simulink library "DQN_Lib (conflicted copy 2023-11-25 154811)"  (R2023b)
settings: Solver=VariableStepAuto  StartTime=0.0  StopTime=10.0  RelTol=1e-3
undefined symbols (not defined in the file): FreqRad, HrmOrd, Init, La, N, R, Ra, TimeStep, Ts, Ts_dqn, Ws
libraries: $bdroot x4, spsMeanVariableFrequencyLib x4, eeTransforms x3, spsabctodq0Lib x2, spsAlphaBetaZerotodq0Lib x1
(part 2 of 8)

== system DQN_Lib (conflicted copy 2023-11-25 154811)/Int_DQN ==
  X_DQN : Inport
  Demux : Demux  Outputs=6
  Int_d_2N_2 : MATLAB Function  TreatAsAtomicUnit=on  mask{N=HrmOrd, dt=TimeStep, w=FreqRad, EMT=EMT, InitInt=Init, chkHrmLst=chkHrmLst, HrmLst=HrmLst}
      mask prompts: N "Order number:"; dt "Time step (s):"; w "Angular frequency (1/rad):"; InitInt "Initial conditions [6x1]:"; chkHrmLst "Only selected harmonics"; HrmLst "Harmonic list:"
  Mux51 : Mux  Inputs=[(1)*HrmOrd+1,(1)*HrmOrd+1,(1)*HrmOrd+1,(1)*HrmOrd+1,(1)*HrmOrd+1,(1)*HrmOrd+1]
  Z_DQN : Outport
  wires:
  X_DQN/1 -> Demux/1
  Mux51/1 -> Z_DQN/1
  Demux/3 -> Int_d_2N_2/3(Xdz)
  Demux/2 -> Int_d_2N_2/2(Xdn)
  Demux/4 -> Int_d_2N_2/4(Xqp)
  Demux/1 -> Int_d_2N_2/1(Xdp)
  Demux/5 -> Int_d_2N_2/5(Xqn)
  Demux/6 -> Int_d_2N_2/6(Xqz)
  Int_d_2N_2/3(Zdz) -> Mux51/3
  Int_d_2N_2/2(Zdn) -> Mux51/2
  Int_d_2N_2/4(Zqp) -> Mux51/4
  Int_d_2N_2/1(Zdp) -> Mux51/1
  Int_d_2N_2/5(Zqn) -> Mux51/5
  Int_d_2N_2/6(Zqz) -> Mux51/6

== system DQN_Lib (conflicted copy 2023-11-25 154811)/Int_DQN_fdbk ==
  X_DQN : Inport
  Demux : Demux  Outputs=6
  Int_d_2N_2 : MATLAB Function  TreatAsAtomicUnit=on  mask{N=HrmOrd, dt=TimeStep, w=FreqRad, SW=swFeed, R=R, iL=iL}
      mask prompts: N "Order number:"; dt "Time step (s):"; w "Angular frequency (1/rad):"; SW "Enable feedback"; R "Feedback parameter (Kr):"; iL "Integrator parameter (Kl):"
  Mux51 : Mux  Inputs=[(1)*HrmOrd+1,(1)*HrmOrd+1,(1)*HrmOrd+1,(1)*HrmOrd+1,(1)*HrmOrd+1,(1)*HrmOrd+1]
  Z_DQN : Outport
  wires:
  Int_d_2N_2/6(Zqz) -> Mux51/6
  Int_d_2N_2/5(Zqn) -> Mux51/5
  Int_d_2N_2/1(Zdp) -> Mux51/1
  Int_d_2N_2/4(Zqp) -> Mux51/4
  Int_d_2N_2/2(Zdn) -> Mux51/2
  Int_d_2N_2/3(Zdz) -> Mux51/3
  Demux/6 -> Int_d_2N_2/6(Xqz)
  Demux/5 -> Int_d_2N_2/5(Xqn)
  Demux/1 -> Int_d_2N_2/1(Xdp)
  Demux/4 -> Int_d_2N_2/4(Xqp)
  Demux/2 -> Int_d_2N_2/2(Xdn)
  Demux/3 -> Int_d_2N_2/3(Xdz)
  Mux51/1 -> Z_DQN/1
  X_DQN/1 -> Demux/1

== system DQN_Lib (conflicted copy 2023-11-25 154811)/MatDemux ==
  In1 : Inport
  Sel1 : Selector  NumberOfDimensions=2  InputPortWidth=3  IndexOptions=Select all,Index vector (dialog)  Indices=1,1:6  OutputSizes=1
  Sel2 : Selector  NumberOfDimensions=2  InputPortWidth=3  IndexOptions=Select all,Index vector (dialog)  Indices=1,7:12  OutputSizes=1
  Sel3 : Selector  NumberOfDimensions=2  InputPortWidth=3  IndexOptions=Select all,Index vector (dialog)  Indices=1,13:18  OutputSizes=1
  Out1 : Outport
  Out2 : Outport  Port=2
  Out3 : Outport  Port=3
  wires:
  In1/1 -> Sel1/1, Sel2/1, Sel3/1
  Sel1/1 -> Out1/1
  Sel2/1 -> Out2/1
  Sel3/1 -> Out3/1

== system DQN_Lib (conflicted copy 2023-11-25 154811)/MatMux ==
  In1 : Inport
  In2 : Inport  Port=2
  In3 : Inport  Port=3
  Mux : Concatenate  NumInputs=3  Mode=Multidimensional array  ConcatenateDimension=2
  Out1 : Outport
  wires:
  In1/1 -> Mux/1
  In2/1 -> Mux/2
  In3/1 -> Mux/3
  Mux/1 -> Out1/1

== system DQN_Lib (conflicted copy 2023-11-25 154811)/Mult_DQN ==
  X_DQN : Inport
  Y_DQN : Inport  Port=2
  DQn (Full)10 : MATLAB Function  TreatAsAtomicUnit=on  mask{N=HrmOrd, HrmDbl=HrmDbl, chkHrmLst=chkHrmLst, HrmLstX=HrmLstX, HrmLstY=HrmLstY}
      mask prompts: N "Harmonic order:"; HrmDbl "Double Harmonic"; chkHrmLst "Only specific harmonics:"; HrmLstX "Harmonic list X:"; HrmLstY "Harmonic list Y:"
  Demux : Demux  Outputs=6
  Demux1 : Demux  Outputs=6
  Mux51 : Mux  Inputs=[(HrmDbl+1)*HrmOrd+1,(HrmDbl+1)*HrmOrd+1,(HrmDbl+1)*HrmOrd+1,(HrmDbl+1)*HrmOrd+1,(HrmDbl+1)*HrmOrd+1,(HrmDbl+1)*HrmOrd+1]
  Z_DQN : Outport
  wires:
  X_DQN/1 -> Demux/1
  Y_DQN/1 -> Demux1/1
  Mux51/1 -> Z_DQN/1
  Demux/1 -> DQn (Full)10/1(Xdp)
  Demux/2 -> DQn (Full)10/2(Xdn)
  Demux/3 -> DQn (Full)10/3(Xdz)
  Demux/4 -> DQn (Full)10/4(Xqp)
  Demux/5 -> DQn (Full)10/5(Xqn)
  Demux/6 -> DQn (Full)10/6(Xqz)
  Demux1/1 -> DQn (Full)10/7(Ydp)
  Demux1/2 -> DQn (Full)10/8(Ydn)
  Demux1/3 -> DQn (Full)10/9(Ydz)
  Demux1/4 -> DQn (Full)10/10(Yqp)
  Demux1/5 -> DQn (Full)10/11(Yqn)
  Demux1/6 -> DQn (Full)10/12(Yqz)
  DQn (Full)10/3(Zdz) -> Mux51/3
  DQn (Full)10/2(Zdn) -> Mux51/2
  DQn (Full)10/4(Zqp) -> Mux51/4
  DQn (Full)10/1(Zdp) -> Mux51/1
  DQn (Full)10/5(Zqn) -> Mux51/5
  DQn (Full)10/6(Zqz) -> Mux51/6

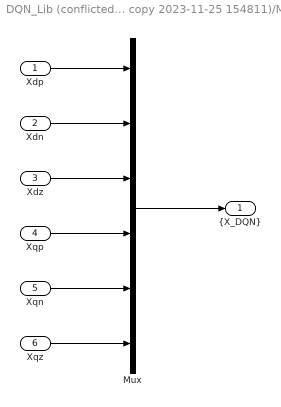
== system DQN_Lib (conflicted copy 2023-11-25 154811)/Mux ==
  Xdp : Inport
  Xdn : Inport  Port=2
  Xdz : Inport  Port=3
  Xqp : Inport  Port=4
  Xqn : Inport  Port=5
  Xqz : Inport  Port=6
  Mux : Mux  Inputs=[N+1, N+1, N+1, N+1, N+1, N+1]
  "{X_DQN}" : Outport
  wires:
  Mux/1 -> "{X_DQN}"/1
  Xdp/1 -> Mux/1
  Xdn/1 -> Mux/2
  Xdz/1 -> Mux/3
  Xqp/1 -> Mux/4
  Xqn/1 -> Mux/5
  Xqz/1 -> Mux/6

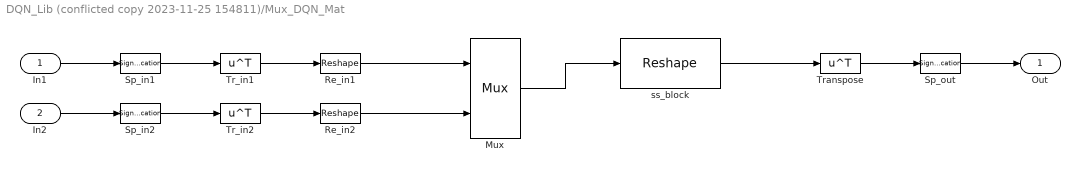
== system DQN_Lib (conflicted copy 2023-11-25 154811)/Mux_DQN_Mat ==
  In1 : Inport
  In2 : Inport  Port=2
  Mux : Mux  Inputs=[6,6]
  Re_in1 : Reshape
  Re_in2 : Reshape
  Sp_in1 : SignalSpecification  Dimensions=[1,6]
  Sp_in2 : SignalSpecification  Dimensions=[1,6]
  Sp_out : SignalSpecification  Dimensions=[2,6]
  Tr_in1 : Math  Operator=transpose
  Tr_in2 : Math  Operator=transpose
  Transpose : Math  Operator=transpose
  ss_block : Reshape  OutputDimensionality=Customize  OutputDimensions=[6,2*(1)]
  Out : Outport
  wires:
  In1/1 -> Sp_in1/1
  Sp_in1/1 -> Tr_in1/1
  Tr_in1/1 -> Re_in1/1
  Re_in1/1 -> Mux/1
  In2/1 -> Sp_in2/1
  Sp_in2/1 -> Tr_in2/1
  Tr_in2/1 -> Re_in2/1
  Re_in2/1 -> Mux/2
  Mux/1 -> ss_block/1
  ss_block/1 -> Transpose/1
  Transpose/1 -> Sp_out/1
  Sp_out/1 -> Out/1

== system DQN_Lib (conflicted copy 2023-11-25 154811)/Mux_DQNc_Mat ==
  In1 : Inport
  In2 : Inport  Port=2
  Mux : Concatenate  Mode=Multidimensional array
  Out1 : Outport
  wires:
  In1/1 -> Mux/1
  In2/1 -> Mux/2
  Mux/1 -> Out1/1

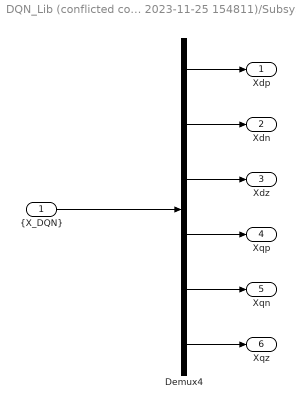
== system DQN_Lib (conflicted copy 2023-11-25 154811)/Subsystem ==
  "{X_DQN}" : Inport
  Demux4 : Demux  Outputs=[N+1, N+1, N+1, N+1, N+1, N+1]
  Xdp : Outport
  Xdn : Outport  Port=2
  Xdz : Outport  Port=3
  Xqp : Outport  Port=4
  Xqn : Outport  Port=5
  Xqz : Outport  Port=6
  wires:
  "{X_DQN}"/1 -> Demux4/1
  Demux4/1 -> Xdp/1
  Demux4/2 -> Xdn/1
  Demux4/3 -> Xdz/1
  Demux4/4 -> Xqp/1
  Demux4/5 -> Xqn/1
  Demux4/6 -> Xqz/1

== system DQN_Lib (conflicted copy 2023-11-25 154811)/Subsystem1 ==
  abc : Inport
  th : Inport  Port=2
  DQN Mux : MATLAB Function  TreatAsAtomicUnit=on  mask{N=1}
      mask prompts: N "Harmonic order:"
  Mux : Mux  Inputs=[1, 1, 1, 1, 1, 1]
  Mux1 : Mux  Inputs=2
  abc-->DQN : $bdroot/abc-->DQN  H=HrmOrd  f=Freq  Ts=Ts
  DQN : Outport
  wires:
  th/1 -> abc-->DQN/2
  abc/1 -> abc-->DQN/1
  abc-->DQN/2 -> Mux/1
  abc-->DQN/3 -> Mux/2
  abc-->DQN/4 -> Mux/3
  abc-->DQN/5 -> Mux/4
  abc-->DQN/6 -> Mux/5
  abc-->DQN/7 -> Mux/6
  DQN Mux/1(y) -> DQN/1
  abc-->DQN/1 -> Mux1/1
  Mux1/1 -> DQN Mux/1(u)
  Mux/1 -> Mux1/2

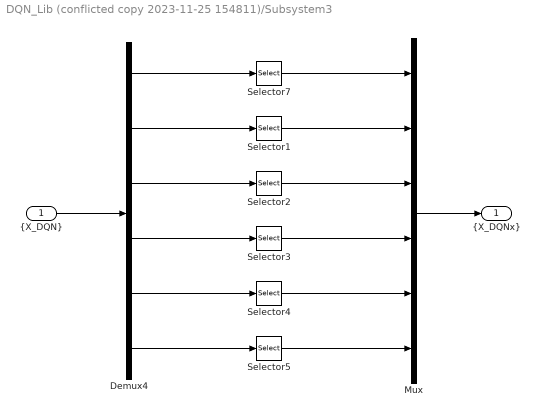
== system DQN_Lib (conflicted copy 2023-11-25 154811)/Subsystem3 ==
  "{X_DQN}" : Inport
  Demux4 : Demux  Outputs=[HOI+1,HOI+1,HOI+1,HOI+1,HOI+1,HOI+1]
  Mux : Mux  Inputs=[HOO+1,HOO+1,HOO+1,HOO+1,HOO+1,HOO+1]
  Selector{1..5,7} (6 alike) : Selector  InputPortWidth=HOI+1  IndexOptions=Index vector (dialog)  Indices=[1:HOO+1]  OutputSizes=1
  "{X_DQNx}" : Outport
  wires:
  "{X_DQN}"/1 -> Demux4/1
  Mux/1 -> "{X_DQNx}"/1
  Selector7/1 -> Mux/1
  Demux4/1 -> Selector7/1
  Selector1/1 -> Mux/2
  Demux4/2 -> Selector1/1
  Demux4/3 -> Selector2/1
  Selector2/1 -> Mux/3
  Demux4/4 -> Selector3/1
  Selector3/1 -> Mux/4
  Demux4/5 -> Selector4/1
  Selector4/1 -> Mux/5
  Demux4/6 -> Selector5/1
  Selector5/1 -> Mux/6

== system DQN_Lib (conflicted copy 2023-11-25 154811)/Subsystem4 ==
  In1 : Inport
  In2 : Inport  Port=2
  Demux : Demux  Outputs=6
  S-Function : S-Function  FunctionName=sDQNabc  SFunctionDeploymentMode=off  EnableBusSupport=off
  Out1 : Outport
  wires:
  Demux/5 -> S-Function/5
  Demux/4 -> S-Function/4
  Demux/6 -> S-Function/6
  Demux/2 -> S-Function/2
  S-Function/1 -> Out1/1
  Demux/1 -> S-Function/1
  Demux/3 -> S-Function/3
  In2/1 -> S-Function/7
  In1/1 -> Demux/1

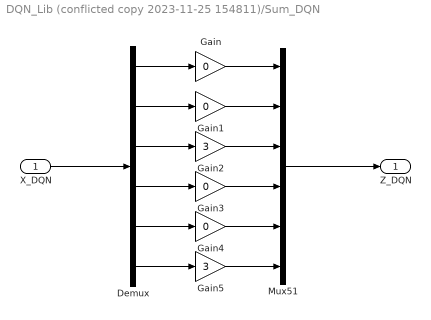
== system DQN_Lib (conflicted copy 2023-11-25 154811)/Sum_DQN ==
  X_DQN : Inport
  Demux : Demux  Outputs=[(1)*HrmOrd+1,(1)*HrmOrd+1,(1)*HrmOrd+1,(1)*HrmOrd+1,(1)*HrmOrd+1,(1)*HrmOrd+1]
  Gain{,1,3..4} (4 alike) : Gain  Gain=0
  Gain2 : Gain  Gain=3
  Gain5 : Gain  Gain=3
  Mux51 : Mux  Inputs=[(1)*HrmOrd+1,(1)*HrmOrd+1,(1)*HrmOrd+1,(1)*HrmOrd+1,(1)*HrmOrd+1,(1)*HrmOrd+1]
  Z_DQN : Outport
  wires:
  Mux51/1 -> Z_DQN/1
  X_DQN/1 -> Demux/1
  Gain/1 -> Mux51/1
  Demux/1 -> Gain/1
  Demux/2 -> Gain1/1
  Gain1/1 -> Mux51/2
  Demux/4 -> Gain3/1
  Demux/5 -> Gain4/1
  Gain4/1 -> Mux51/5
  Gain3/1 -> Mux51/4
  Demux/3 -> Gain2/1
  Gain2/1 -> Mux51/3
  Demux/6 -> Gain5/1
  Gain5/1 -> Mux51/6

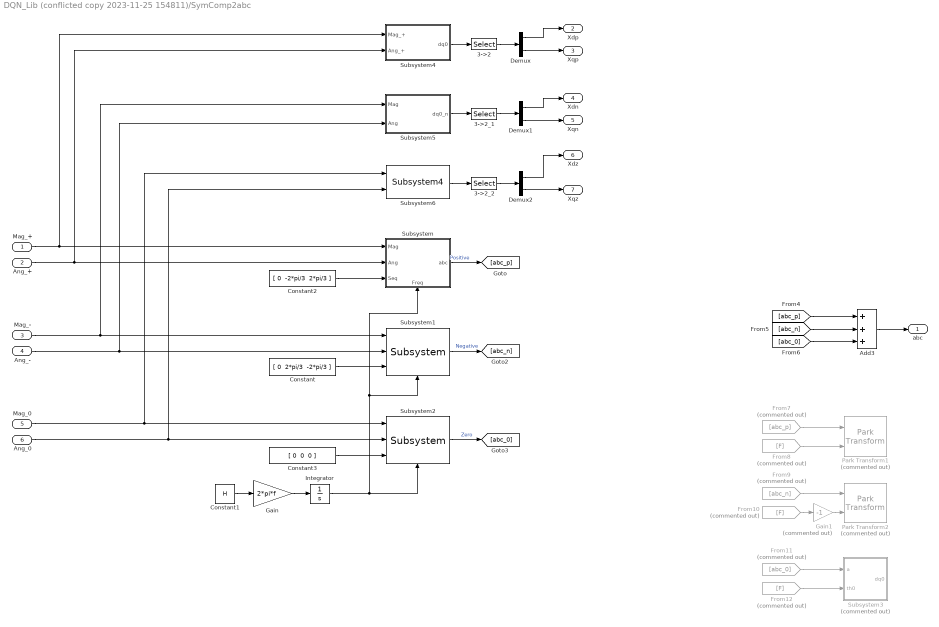
== system DQN_Lib (conflicted copy 2023-11-25 154811)/SymComp2abc ==
  Mag_+ : Inport
  Ang_+ : Inport  Port=2
  Mag_- : Inport  Port=3
  Ang_- : Inport  Port=4
  Mag_0 : Inport  Port=5
  Ang_0 : Inport  Port=6
  3->2 : Selector  InputPortWidth=3  IndexOptions=Index vector (dialog)  Indices=[1 2]  OutputSizes=1
  3->2_1 : Selector  InputPortWidth=3  IndexOptions=Index vector (dialog)  Indices=[1 2]  OutputSizes=1
  3->2_2 : Selector  InputPortWidth=3  IndexOptions=Index vector (dialog)  Indices=[1 2]  OutputSizes=1
  Add3 : Sum  Inputs=+++
  Constant : Constant  Value="[ 0  2*pi/3  -2*pi/3 ]"  SampleTime=-1
  Constant1 : Constant  Value=H
  Constant2 : Constant  Value="[ 0  -2*pi/3  2*pi/3 ]"  SampleTime=-1
  Constant3 : Constant  Value="[ 0  0  0 ]"  SampleTime=-1
  Demux : Demux  Outputs=2
  Demux1 : Demux  Outputs=2
  Demux2 : Demux  Outputs=2
  From10 : From  Commented=on  GotoTag=F  TagVisibility=global
  From11 : From  Commented=on  GotoTag=abc_0
  From12 : From  Commented=on  GotoTag=F  TagVisibility=global
  From7 : From  Commented=on  GotoTag=abc_p
  From8 : From  Commented=on  GotoTag=F  TagVisibility=global
  From9 : From  Commented=on  GotoTag=abc_n
  Gain : Gain  Gain=2*pi*f
  Gain1 : Gain  Commented=on  Gain=-1
  Integrator : Integrator
  Park Transform1 : eeTransforms/Park Transform  Commented=on  AxisAlignment=Q-axis  PowerInvariant=off
  Park Transform2 : eeTransforms/Park Transform  Commented=on  AxisAlignment=Q-axis  PowerInvariant=off
  Subsystem : Subsystem
      settings: PortSchema="{\"entries\":[{\"content\":{\"sides\":[{\"content\":{\"connectorIds\":[\"In1\",\"In2\",\"In3\"]},\"type\":\"ConnectorPlacement.EquallySpacedRectSide\",\"uuid\":\"5249a1eb-6a19-45ae-a6c1-58d43d0bf9b3\"},{\"content\":{\"connectorIds\":[\"Out1\"],\"side\":\"RIGHT\"},\"type\":\"ConnectorPlacement.EquallySpacedRectSide\",\"uuid\":\"d325c733-420b-4f5f-9ace-c19b00cf8826\"},{\"content\":{\"connectorIds\":[],\"side\":\"TOP\"},\"type\":\"ConnectorPlacement.EquallySpacedRectSide\",\"uuid\":\"60868f6e-0774-4fe1-9db3-1bee308f48b3\"},{\"content\":{\"connectorIds\":[\"In4\"],\"side\":\"BOTTOM\"},\"type\":\"ConnectorPlacement.EquallySpacedRectSide\",\"uuid\":\"80f0de2d-2670-46ac-8be7-cd51553925e9\"}]},\"type\":\"ConnectorPlacement.EquallySpacedConnector\",\"uuid\":\"54bcfdba-c1b3-49d1-92ea-2e44c911d179\"}],\"packageUris\":[\"http://schema.mathworks.com/mf0/Connector/R2020b\"],\"version\":\"1.0\"}"
  Subsystem1 : $bdroot/SymComp2abc/Subsystem  SystemSampleTime=-1  VariantActivationTime=update diagram  AllowFlexibleInterface=on  Latency=0  AutoFrameSizeCalculation=off
      settings: PortSchema="{\"entries\":[{\"content\":{\"sides\":[{\"content\":{\"connectorIds\":[\"In1\",\"In2\",\"In3\"]},\"type\":\"ConnectorPlacement.EquallySpacedRectSide\",\"uuid\":\"5249a1eb-6a19-45ae-a6c1-58d43d0bf9b3\"},{\"content\":{\"connectorIds\":[\"Out1\"],\"side\":\"RIGHT\"},\"type\":\"ConnectorPlacement.EquallySpacedRectSide\",\"uuid\":\"d325c733-420b-4f5f-9ace-c19b00cf8826\"},{\"content\":{\"connectorIds\":[],\"side\":\"TOP\"},\"type\":\"ConnectorPlacement.EquallySpacedRectSide\",\"uuid\":\"60868f6e-0774-4fe1-9db3-1bee308f48b3\"},{\"content\":{\"connectorIds\":[\"In4\"],\"side\":\"BOTTOM\"},\"type\":\"ConnectorPlacement.EquallySpacedRectSide\",\"uuid\":\"80f0de2d-2670-46ac-8be7-cd51553925e9\"}]},\"type\":\"ConnectorPlacement.EquallySpacedConnector\",\"uuid\":\"54bcfdba-c1b3-49d1-92ea-2e44c911d179\"}],\"packageUris\":[\"http://schema.mathworks.com/mf0/Connector/R2020b\"],\"version\":\"1.0\"}"
  Subsystem2 : $bdroot/SymComp2abc/Subsystem  SystemSampleTime=-1  VariantActivationTime=update diagram  AllowFlexibleInterface=on  Latency=0  AutoFrameSizeCalculation=off
      settings: PortSchema="{\"entries\":[{\"content\":{\"sides\":[{\"content\":{\"connectorIds\":[\"In1\",\"In2\",\"In3\"]},\"type\":\"ConnectorPlacement.EquallySpacedRectSide\",\"uuid\":\"5249a1eb-6a19-45ae-a6c1-58d43d0bf9b3\"},{\"content\":{\"connectorIds\":[\"Out1\"],\"side\":\"RIGHT\"},\"type\":\"ConnectorPlacement.EquallySpacedRectSide\",\"uuid\":\"d325c733-420b-4f5f-9ace-c19b00cf8826\"},{\"content\":{\"connectorIds\":[],\"side\":\"TOP\"},\"type\":\"ConnectorPlacement.EquallySpacedRectSide\",\"uuid\":\"60868f6e-0774-4fe1-9db3-1bee308f48b3\"},{\"content\":{\"connectorIds\":[\"In4\"],\"side\":\"BOTTOM\"},\"type\":\"ConnectorPlacement.EquallySpacedRectSide\",\"uuid\":\"80f0de2d-2670-46ac-8be7-cd51553925e9\"}]},\"type\":\"ConnectorPlacement.EquallySpacedConnector\",\"uuid\":\"54bcfdba-c1b3-49d1-92ea-2e44c911d179\"}],\"packageUris\":[\"http://schema.mathworks.com/mf0/Connector/R2020b\"],\"version\":\"1.0\"}"
  Subsystem3 : Subsystem  Commented=on
  Subsystem4 : Subsystem
  Subsystem5 : Subsystem
  Subsystem6 : $bdroot/SymComp2abc/Subsystem4  SystemSampleTime=-1  VariantActivationTime=update diagram  AllowFlexibleInterface=on  Latency=0  AutoFrameSizeCalculation=off
  abc : Outport
  Xdp : Outport  Port=2
  Xqp : Outport  Port=3
  Xdn : Outport  Port=4
  Xqn : Outport  Port=5
  Xdz : Outport  Port=6
  Xqz : Outport  Port=7
  wires:
  Constant3/1 -> Subsystem2/3
  Add3/1 -> abc/1
  Mag_-/1 -> Subsystem1/1, Subsystem5/1(Mag)
  Ang_+/1 -> Subsystem/2(Ang), Subsystem4/2(Ang_+)
  From11/1 -> Subsystem3/1(a)
  Mag_0/1 -> Subsystem6/1, Subsystem2/1
  Gain/1 -> Integrator/1
  From12/1 -> Subsystem3/2(th0)
  Subsystem/1(abc) -> [abc_p]  "Positive"
  Constant/1 -> Subsystem1/3
  Gain1/1 -> Park Transform2/2
  [abc_n] -> Add3/2
  From9/1 -> Park Transform2/1
  Ang_-/1 -> Subsystem1/2, Subsystem5/2(Ang)
  From8/1 -> Park Transform1/2
  Constant1/1 -> Gain/1
  Subsystem2/1 -> [abc_0]  "Zero"
  [abc_p] -> Add3/1
  Subsystem1/1 -> [abc_n]  "Negative"
  Ang_0/1 -> Subsystem6/2, Subsystem2/2
  [abc_0] -> Add3/3
  From10/1 -> Gain1/1
  Mag_+/1 -> Subsystem/1(Mag), Subsystem4/1(Mag_+)
  Constant2/1 -> Subsystem/3(Seq)
  From7/1 -> Park Transform1/1
  Integrator/1 -> Subsystem2/4, Subsystem1/4, Subsystem/4(Freq)
  Subsystem4/1(dq0) -> 3->2/1
  3->2/1 -> Demux/1
  3->2_1/1 -> Demux1/1
  Subsystem5/1(dq0_n) -> 3->2_1/1
  Subsystem6/1 -> 3->2_2/1
  3->2_2/1 -> Demux2/1
  Demux/1 -> Xdp/1
  Demux/2 -> Xqp/1
  Demux1/1 -> Xdn/1
  Demux1/2 -> Xqn/1
  Demux2/1 -> Xdz/1
  Demux2/2 -> Xqz/1

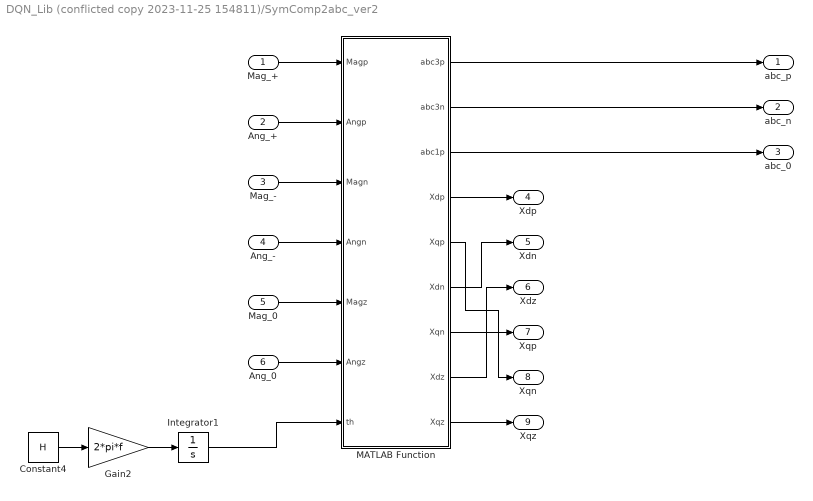
== system DQN_Lib (conflicted copy 2023-11-25 154811)/SymComp2abc_ver2 ==
  Mag_+ : Inport
  Ang_+ : Inport  Port=2
  Mag_- : Inport  Port=3
  Ang_- : Inport  Port=4
  Mag_0 : Inport  Port=5
  Ang_0 : Inport  Port=6
  Constant4 : Constant  Value=H
  Gain2 : Gain  Gain=2*pi*f
  Integrator1 : Integrator
  MATLAB Function : MATLAB Function  TreatAsAtomicUnit=on
  abc_p : Outport
  abc_n : Outport  Port=2
  abc_0 : Outport  Port=3
  Xdp : Outport  Port=4
  Xdn : Outport  Port=5
  Xdz : Outport  Port=6
  Xqp : Outport  Port=7
  Xqn : Outport  Port=8
  Xqz : Outport  Port=9
  wires:
  Mag_-/1 -> MATLAB Function/3(Magn)
  Ang_+/1 -> MATLAB Function/2(Angp)
  Mag_+/1 -> MATLAB Function/1(Magp)
  Ang_-/1 -> MATLAB Function/4(Angn)
  Mag_0/1 -> MATLAB Function/5(Magz)
  Ang_0/1 -> MATLAB Function/6(Angz)
  Gain2/1 -> Integrator1/1
  Constant4/1 -> Gain2/1
  Integrator1/1 -> MATLAB Function/7(th)
  MATLAB Function/4(Xdp) -> Xdp/1
  MATLAB Function/7(Xqn) -> Xqn/1
  MATLAB Function/8(Xdz) -> Xdz/1
  MATLAB Function/6(Xdn) -> Xdn/1
  MATLAB Function/5(Xqp) -> Xqp/1
  MATLAB Function/9(Xqz) -> Xqz/1
  MATLAB Function/1(abc3p) -> abc_p/1
  MATLAB Function/2(abc3n) -> abc_n/1
  MATLAB Function/3(abc1p) -> abc_0/1

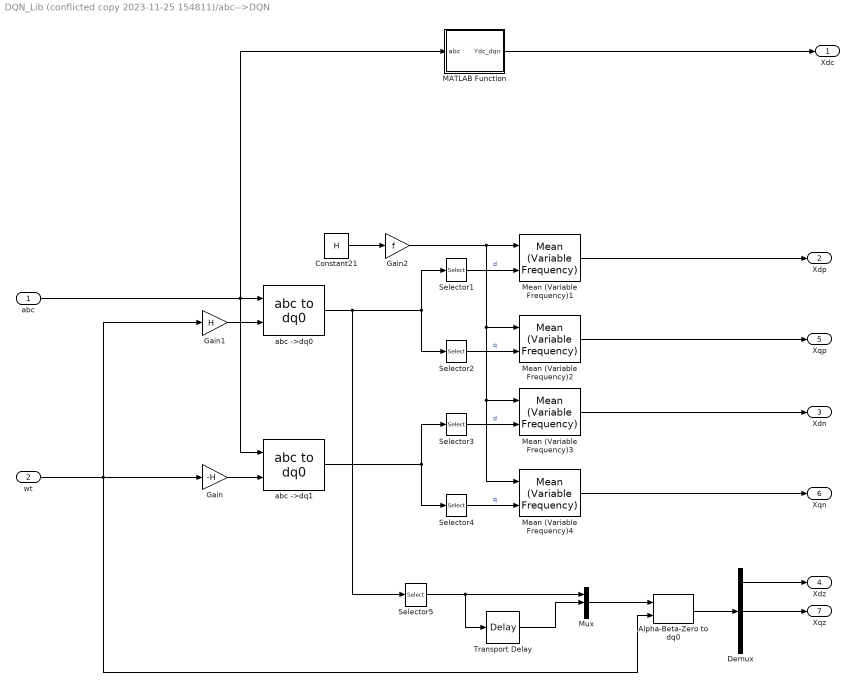
== system DQN_Lib (conflicted copy 2023-11-25 154811)/abc-->DQN ==
  abc : Inport
  wt : Inport  Port=2
  Alpha-Beta-Zero to dq0 : spsAlphaBetaZerotodq0Lib/Alpha-Beta-Zero to dq0  Alignment=90 degrees behind phase A axis
  Constant21 : Constant  Value=H
  Demux : Demux  Outputs=3
  Gain : Gain  Gain=-H
  Gain1 : Gain  Gain=H
  Gain2 : Gain  Gain=f
  MATLAB Function : MATLAB Function  TreatAsAtomicUnit=on
  Mean (Variable Frequency){1..4} (4 alike) : spsMeanVariableFrequencyLib/Mean (Variable Frequency)  Finit=50  Fmin=45  Vinit=0  Ts=Ts
  Mux : Mux  Inputs=3
  Selector1 : Selector  InputPortWidth=3  IndexOptions=Index vector (dialog)  Indices=[1]  OutputSizes=1
  Selector2 : Selector  InputPortWidth=3  IndexOptions=Index vector (dialog)  Indices=[2]  OutputSizes=1
  Selector3 : Selector  InputPortWidth=3  IndexOptions=Index vector (dialog)  Indices=[1]  OutputSizes=1
  Selector4 : Selector  InputPortWidth=3  IndexOptions=Index vector (dialog)  Indices=[2]  OutputSizes=1
  Selector5 : Selector  InputPortWidth=3  IndexOptions=Index vector (dialog)  Indices=[3]  OutputSizes=1
  Transport Delay : TransportDelay  DelayTime=(90/360)*1/(H*f)
  abc ->dq0 : spsabctodq0Lib/abc to dq0  Alignment=90 degrees behind phase A axis
  abc ->dq1 : spsabctodq0Lib/abc to dq0  Alignment=90 degrees behind phase A axis
  Xdc : Outport
  Xdp : Outport  Port=2
  Xdn : Outport  Port=3
  Xdz : Outport  Port=4
  Xqp : Outport  Port=5
  Xqn : Outport  Port=6
  Xqz : Outport  Port=7
  wires:
  Selector3/1 -> Mean (Variable Frequency)3/2  "d"
  abc ->dq1/1 -> Selector3/1, Selector4/1
  Gain2/1 -> Mean (Variable Frequency)2/1, Mean (Variable Frequency)3/1, Mean (Variable Frequency)4/1, Mean (Variable Frequency)1/1
  Selector1/1 -> Mean (Variable Frequency)1/2  "d"
  abc ->dq0/1 -> Selector5/1, Selector1/1, Selector2/1
  Selector4/1 -> Mean (Variable Frequency)4/2  "q"
  Selector2/1 -> Mean (Variable Frequency)2/2  "q"
  Mean (Variable Frequency)3/1 -> Xdn/1
  Mean (Variable Frequency)2/1 -> Xqp/1
  Mean (Variable Frequency)1/1 -> Xdp/1
  Mean (Variable Frequency)4/1 -> Xqn/1
  wt/1 -> Gain/1, Alpha-Beta-Zero to dq0/2, Gain1/1
  abc/1 -> MATLAB Function/1(abc), abc ->dq1/1, abc ->dq0/1
  Selector5/1 -> Transport Delay/1, Mux/1
  Transport Delay/1 -> Mux/2
  Mux/1 -> Alpha-Beta-Zero to dq0/1
  Alpha-Beta-Zero to dq0/1 -> Demux/1
  Demux/1 -> Xdz/1
  Demux/2 -> Xqz/1
  Gain/1 -> abc ->dq1/2
  Gain1/1 -> abc ->dq0/2
  Constant21/1 -> Gain2/1
  MATLAB Function/1(Ydc_dqn) -> Xdc/1

== system DQN_Lib (conflicted copy 2023-11-25 154811)/sAdd_DQN ==
  In1 : Inport
  In2 : Inport  Port=2
  Demux : Demux  Outputs=6
  Demux7 : Demux  Outputs=6
  Mux7 : Mux  Inputs=[HRM+1,HRM+1,HRM+1,HRM+1,HRM+1,HRM+1]
  S-Function : S-Function  FunctionName=sAddDQN  Parameters=HRM  SFunctionDeploymentMode=off  EnableBusSupport=off  mask{HRM=HRM}
      mask prompts: HRM "Harmonic order:"
  Out1 : Outport
  wires:
  S-Function/6 -> Mux7/6
  S-Function/4 -> Mux7/4
  S-Function/3 -> Mux7/3
  Demux7/5 -> S-Function/11
  S-Function/5 -> Mux7/5
  S-Function/1 -> Mux7/1
  Demux/3 -> S-Function/3
  S-Function/2 -> Mux7/2
  Demux/2 -> S-Function/2
  In2/1 -> Demux7/1
  Demux/6 -> S-Function/6
  Mux7/1 -> Out1/1
  Demux7/3 -> S-Function/9
  Demux/4 -> S-Function/4
  Demux7/1 -> S-Function/7
  Demux7/4 -> S-Function/10
  Demux/5 -> S-Function/5
  Demux7/6 -> S-Function/12
  Demux7/2 -> S-Function/8
  Demux/1 -> S-Function/1
  In1/1 -> Demux/1

== system DQN_Lib (conflicted copy 2023-11-25 154811)/sDQN2abc ==
  "{DQN}" : Inport
  th : Inport  Port=2
  Demux : Demux  Outputs=6
  S-Function : S-Function  FunctionName=sDQNabcN  Parameters=HRM  SFunctionDeploymentMode=off  EnableBusSupport=off
  abc : Outport
  wires:
  S-Function/1 -> abc/1
  th/1 -> S-Function/7
  Demux/1 -> S-Function/1
  Demux/2 -> S-Function/2
  Demux/3 -> S-Function/3
  Demux/4 -> S-Function/4
  Demux/5 -> S-Function/5
  Demux/6 -> S-Function/6
  "{DQN}"/1 -> Demux/1

== system DQN_Lib (conflicted copy 2023-11-25 154811)/sInt_DQN ==
  In1 : Inport
  Demux : Demux  Outputs=[HRM+1,HRM+1,HRM+1,HRM+1,HRM+1,HRM+1]
  Mux1 : Mux  Inputs=[HRM+1,HRM+1,HRM+1,HRM+1,HRM+1,HRM+1]
  S-Function : S-Function  FunctionName=sIntDQN  Parameters=HRM Ts Ws HrmSeq  SFunctionDeploymentMode=off  EnableBusSupport=off
  Out1 : Outport
  wires:
  Demux/3 -> S-Function/3
  S-Function/1 -> Mux1/1
  Demux/6 -> S-Function/6
  Demux/2 -> S-Function/2
  Demux/1 -> S-Function/1
  Demux/5 -> S-Function/5
  S-Function/6 -> Mux1/6
  Demux/4 -> S-Function/4
  S-Function/4 -> Mux1/4
  S-Function/2 -> Mux1/2
  S-Function/5 -> Mux1/5
  S-Function/3 -> Mux1/3
  In1/1 -> Demux/1
  Mux1/1 -> Out1/1

== system DQN_Lib (conflicted copy 2023-11-25 154811)/sInt_DQN_fdbk ==
  In1 : Inport
  Demux : Demux  Outputs=[HRM+1,HRM+1,HRM+1,HRM+1,HRM+1,HRM+1]
  Mux1 : Mux  Inputs=[HRM+1,HRM+1,HRM+1,HRM+1,HRM+1,HRM+1]
  S-Function : S-Function  FunctionName=sIntDQNfdbk  Parameters=HRM Ts Ws HrmSeq swFeed R iL  SFunctionDeploymentMode=off  EnableBusSupport=off
  Out1 : Outport
  wires:
  Mux1/1 -> Out1/1
  In1/1 -> Demux/1
  S-Function/3 -> Mux1/3
  S-Function/5 -> Mux1/5
  S-Function/2 -> Mux1/2
  S-Function/4 -> Mux1/4
  Demux/4 -> S-Function/4
  S-Function/6 -> Mux1/6
  Demux/5 -> S-Function/5
  Demux/1 -> S-Function/1
  Demux/2 -> S-Function/2
  Demux/6 -> S-Function/6
  S-Function/1 -> Mux1/1
  Demux/3 -> S-Function/3

== system DQN_Lib (conflicted copy 2023-11-25 154811)/sMult_DQN ==
  In1 : Inport
  In2 : Inport  Port=2
  Demux : Demux  Outputs=6
  Demux7 : Demux  Outputs=6
  Mux7 : Mux  Inputs=[(HrmDbl+1)*HRM+1,(HrmDbl+1)*HRM+1,(HrmDbl+1)*HRM+1,(HrmDbl+1)*HRM+1,(HrmDbl+1)*HRM+1,(HrmDbl+1)*HRM+1]
  S-Function : S-Function  FunctionName=sMultDQN  Parameters=HRM chkHrm  SFunctionDeploymentMode=off  EnableBusSupport=off  mask{HRM=HRM, chkHrm=HrmOpt}
      mask prompts: HRM "Harmonic order:"; chkHrm "Double harmonic:"
  Out1 : Outport
  wires:
  S-Function/6 -> Mux7/6
  S-Function/4 -> Mux7/4
  S-Function/3 -> Mux7/3
  Demux7/5 -> S-Function/11
  S-Function/5 -> Mux7/5
  S-Function/1 -> Mux7/1
  Demux/3 -> S-Function/3
  S-Function/2 -> Mux7/2
  Demux/2 -> S-Function/2
  In2/1 -> Demux7/1
  Demux/6 -> S-Function/6
  Mux7/1 -> Out1/1
  Demux7/3 -> S-Function/9
  Demux/4 -> S-Function/4
  Demux7/1 -> S-Function/7
  Demux7/4 -> S-Function/10
  Demux/5 -> S-Function/5
  Demux7/6 -> S-Function/12
  Demux7/2 -> S-Function/8
  Demux/1 -> S-Function/1
  In1/1 -> Demux/1

== system DQN_Lib (conflicted copy 2023-11-25 154811)/sMult_DQN2 ==
  In1 : Inport
  In2 : Inport  Port=2
  Demux : Demux  Outputs=6
  Demux7 : Demux  Outputs=6
  Mux7 : Mux  Inputs=[(HrmDbl+1)*HRM+1,(HrmDbl+1)*HRM+1,(HrmDbl+1)*HRM+1,(HrmDbl+1)*HRM+1,(HrmDbl+1)*HRM+1,(HrmDbl+1)*HRM+1]
  S-Function : S-Function  FunctionName=sMultDQN2  Parameters=HRM chkHrm ENH  SFunctionDeploymentMode=off  EnableBusSupport=off  mask{HRM=HRM, chkHrm=HrmOpt, ENH=selMat}
      mask prompts: HRM "Harmonic order:"; chkHrm "Double harmonic:"; ENH "Enabled harmonics (mat):"
  Out1 : Outport
  wires:
  S-Function/6 -> Mux7/6
  S-Function/4 -> Mux7/4
  S-Function/3 -> Mux7/3
  Demux7/5 -> S-Function/11
  S-Function/5 -> Mux7/5
  S-Function/1 -> Mux7/1
  Demux/3 -> S-Function/3
  S-Function/2 -> Mux7/2
  Demux/2 -> S-Function/2
  In2/1 -> Demux7/1
  Demux/6 -> S-Function/6
  Mux7/1 -> Out1/1
  Demux7/3 -> S-Function/9
  Demux/4 -> S-Function/4
  Demux7/1 -> S-Function/7
  Demux7/4 -> S-Function/10
  Demux/5 -> S-Function/5
  Demux7/6 -> S-Function/12
  Demux7/2 -> S-Function/8
  Demux/1 -> S-Function/1
  In1/1 -> Demux/1

== system DQN_Lib (conflicted copy 2023-11-25 154811)/sMult_DQN_old ==
  In1 : Inport
  In2 : Inport  Port=2
  Demux : Demux  Outputs=6
  Demux7 : Demux  Outputs=6
  Mux7 : Mux  Inputs=[(HrmDbl+1)*HrmOrd+1,(HrmDbl+1)*HrmOrd+1,(HrmDbl+1)*HrmOrd+1,(HrmDbl+1)*HrmOrd+1,(HrmDbl+1)*HrmOrd+1,(HrmDbl+1)*HrmOrd+1]
  S-Function : S-Function  FunctionName=sMultDQN  Parameters=HRM  SFunctionDeploymentMode=off  EnableBusSupport=off  mask{HRM=HrmOrd}
      mask prompts: HRM "Harmonic order:"
  Out1 : Outport
  wires:
  S-Function/3 -> Mux7/3
  S-Function/2 -> Mux7/2
  Demux7/5 -> S-Function/11
  Demux/5 -> S-Function/5
  Demux/3 -> S-Function/3
  Demux7/1 -> S-Function/7
  Demux/6 -> S-Function/6
  Demux/1 -> S-Function/1
  Demux/4 -> S-Function/4
  S-Function/4 -> Mux7/4
  Demux7/6 -> S-Function/12
  Demux7/3 -> S-Function/9
  Demux7/2 -> S-Function/8
  Demux7/4 -> S-Function/10
  Demux/2 -> S-Function/2
  S-Function/6 -> Mux7/6
  S-Function/1 -> Mux7/1
  In2/1 -> Demux7/1
  S-Function/5 -> Mux7/5
  In1/1 -> Demux/1
  Mux7/1 -> Out1/1

== system DQN_Lib (conflicted copy 2023-11-25 154811)/sSumDQN ==
  In1 : Inport
  Demux18 : Demux  Outputs=[HrmOrd+1,HrmOrd+1,HrmOrd+1,HrmOrd+1,HrmOrd+1,HrmOrd+1]
  Mux26 : Mux  Inputs=[HrmOrd+1,HrmOrd+1,HrmOrd+1,HrmOrd+1,HrmOrd+1,HrmOrd+1]
  S-Function : S-Function  FunctionName=sSumDQN  Parameters=HrmOrd  SFunctionDeploymentMode=off  EnableBusSupport=off
  Out1 : Outport
  wires:
  S-Function/1 -> Mux26/1  "[(HrmDbl+1)*HRM+1"
  Demux18/3 -> S-Function/3
  Demux18/5 -> S-Function/5
  Demux18/2 -> S-Function/2
  Demux18/4 -> S-Function/4
  S-Function/6 -> Mux26/6  "(HrmDbl+1)*HRM+1]"
  In1/1 -> Demux18/1
  S-Function/2 -> Mux26/2  "(HrmDbl+1)*HRM+1"
  Demux18/6 -> S-Function/6
  S-Function/3 -> Mux26/3  "(HrmDbl+1)*HRM+1"
  Demux18/1 -> S-Function/1
  S-Function/4 -> Mux26/4  "(HrmDbl+1)*HRM+1"
  S-Function/5 -> Mux26/5  "(HrmDbl+1)*HRM+1"
  Mux26/1 -> Out1/1

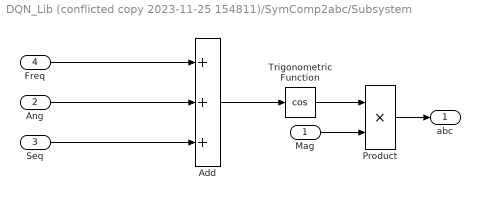
== system DQN_Lib (conflicted copy 2023-11-25 154811)/SymComp2abc/Subsystem ==
  Mag : Inport
  Ang : Inport  Port=2
  Seq : Inport  Port=3
  Freq : Inport  Port=4
  Add : Sum  Inputs=+++
  Product : Product  RndMeth=Zero
  Trigonometric Function : Trigonometry  Operator=cos
  abc : Outport
  wires:
  Add/1 -> Trigonometric Function/1
  Ang/1 -> Add/2
  Trigonometric Function/1 -> Product/1
  Mag/1 -> Product/2
  Seq/1 -> Add/3
  Product/1 -> abc/1
  Freq/1 -> Add/1

== system DQN_Lib (conflicted copy 2023-11-25 154811)/SymComp2abc/Subsystem3 ==
  a : Inport
  th0 : Inport  Port=2
  Clarke to Park Angle Transform : eeTransforms/Clarke to Park Angle Transform  AxisAlignment=Q-axis
  Mux12 : Mux  Inputs=3
  Pi : Constant  Value=0  OutDataTypeStr=Inherit: Inherit via back propagation
  Selector2 : Selector  InputPortWidth=3  IndexOptions=Index vector (dialog)  Indices=[1]  OutputSizes=1
  Transport Delay : TransportDelay  DelayTime=0.005
  dq0 : Outport
  wires:
  th0/1 -> Clarke to Park Angle Transform/2
  Pi/1 -> Mux12/3
  Transport Delay/1 -> Mux12/2
  Mux12/1 -> Clarke to Park Angle Transform/1
  a/1 -> Selector2/1
  Clarke to Park Angle Transform/1 -> dq0/1
  Selector2/1 -> Transport Delay/1, Mux12/1

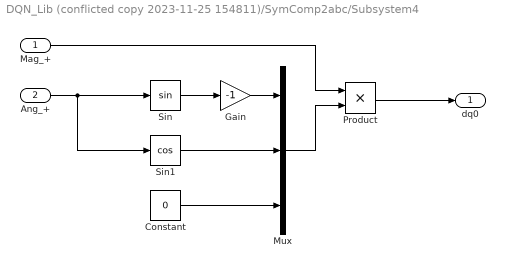
== system DQN_Lib (conflicted copy 2023-11-25 154811)/SymComp2abc/Subsystem4 ==
  Mag_+ : Inport
  Ang_+ : Inport  Port=2
  Constant : Constant  Value=0
  Gain : Gain  Gain=-1
  Mux : Mux  Inputs=3
  Product : Product
  Sin : Trigonometry
  Sin1 : Trigonometry  Operator=cos
  dq0 : Outport
  wires:
  Sin/1 -> Gain/1
  Mux/1 -> Product/2
  Ang_+/1 -> Sin1/1, Sin/1
  Gain/1 -> Mux/1
  Sin1/1 -> Mux/2
  Mag_+/1 -> Product/1
  Product/1 -> dq0/1
  Constant/1 -> Mux/3

== system DQN_Lib (conflicted copy 2023-11-25 154811)/SymComp2abc/Subsystem5 ==
  Mag : Inport
  Ang : Inport  Port=2
  Constant12 : Constant  Value=0
  Mux : Mux  Inputs=3
  Product : Product
  Sin : Trigonometry
  Sin1 : Trigonometry  Operator=cos
  dq0_n : Outport
  wires:
  Mux/1 -> Product/2
  Sin1/1 -> Mux/2
  Ang/1 -> Sin1/1, Sin/1
  Sin/1 -> Mux/1
  Constant12/1 -> Mux/3
  Mag/1 -> Product/1
  Product/1 -> dq0_n/1

== matlab function DQN_Lib (conflicted copy 2023-11-25 154811)/Der_DQN/MATLAB Function3 ==
  settings: updateMethod=DISCRETE
  data: Xdp input; Xdn input; Xdz input; Xqp input; Xqn input; Xqz input; dZdp output; dZdn output; dZdz output; dZqp output; dZqn output; dZqz output; N parameter; w parameter; EMT parameter; Ts parameter; sw_soft parameter; chkHrmLst parameter; HrmLst parameter
function [dZdp,dZdn,dZdz,dZqp,dZqn,dZqz]  = DerDQN(Xdp, Xdn, Xdz, Xqp, Xqn, Xqz, N, w, EMT, Ts, sw_soft, chkHrmLst, HrmLst)   
    
    persistent Xdp_old;
    persistent Xqp_old;
    persistent Xdn_old;
    persistent Xqn_old;
    persistent Xdz_old;
    persistent Xqz_old;
    persistent firstStep;
    persistent HrmLst2;
    
    Xdp = [Xdp(2:end); zeros(N-numel(Xdp)+1,1)];
    Xqp = [Xqp(2:end); zeros(N-numel(Xqp)+1,1)];
    Xdn = [Xdn(2:end); zeros(N-numel(Xdn)+1,1)];
    Xqn = [Xqn(2:end); zeros(N-numel(Xqn)+1,1)];
    Xdz = [Xdz(2:end); zeros(N-numel(Xdz)+1,1)];
    Xqz = [Xqz(2:end); zeros(N-numel(Xqz)+1,1)];
       
    dZdp = zeros(N+1,1);
    dZdn = zeros(N+1,1);
    dZqp = zeros(N+1,1);
    dZqn = zeros(N+1,1);
    dZdz = zeros(N+1,1);
    dZqz = zeros(N+1,1);
    
    if(N>0)
        
        if(isempty(Xdp_old)) 
            Xdp_old  = zeros(N,1); 
            Xqp_old  = zeros(N,1);
            Xdn_old  = zeros(N,1);
            Xqn_old  = zeros(N,1);
            Xdz_old  = zeros(N,1);
            Xqz_old  = zeros(N,1);
            firstStep = 0;
            HrmLst2 = HrmLst;
            HrmLst2(HrmLst2==0) = [];
        end

        if(chkHrmLst)

            range = numel(HrmLst2);
        else
            range = N; 
        end
        
        i = 1;
    
        for g = 1 : range
            
            if(chkHrmLst)
                if(HrmLst2(g)>0)
                    i = HrmLst2(g);
                end
            else
                i = g; 
            end
            
            wn = i*w;
            if(EMT)
                if(sw_soft==1 && firstStep == 0)
                Xdp_old(i) = Xdp(i);
                Xqp_old(i) = Xqp(i);
                Xdn_old(i) = Xdn(i);
                Xqn_old(i) = Xqn(i);
                Xdz_old(i) = Xdz(i);
                Xqz_old(i) = Xqz(i);
                else
                dZdp(i) = (Xdp(i)-Xdp_old(i))/Ts;
                Xdp_old(i) = Xdp(i);
                dZqp(i) = (Xqp(i)-Xqp_old(i))/Ts;
                Xqp_old(i) = Xqp(i);
                dZdn(i) = (Xdn(i)-Xdn_old(i))/Ts;
                Xdn_old(i) = Xdn(i);
                dZqn(i) = (Xqn(i)-Xqn_old(i))/Ts;
                Xqn_old(i) = Xqn(i);
                dZdz(i) = (Xdz(i)-Xdz_old(i))/Ts;
                Xdz_old(i) = Xdz(i);
                dZqz(i) = (Xqz(i)-Xqz_old(i))/Ts;
                Xqz_old(i) = Xqz(i);
                end

            end

            dZdp(i) = dZdp(i) + Xqp(i)*(-(wn));
            dZqp(i) = dZqp(i) + Xdp(i)*((wn)); 

            dZdn(i) = dZdn(i) + Xqn(i)*((wn));
            dZqn(i) = dZqn(i) + Xdn(i)*(-(wn)); 

            dZdz(i) = dZdz(i) + Xqz(i)*(-(wn));
            dZqz(i) = dZqz(i) + Xdz(i)*((wn)); 
        end

        firstStep = 1;

        dZdp(2:end) = dZdp(1:end-1);
        dZqp(2:end) = dZqp(1:end-1);
        dZdn(2:end) = dZdn(1:end-1);
        dZqn(2:end) = dZqn(1:end-1);
        dZdz(2:end) = dZdz(1:end-1);
        dZqz(2:end) = dZqz(1:end-1);
    
    end
    dZdp(1)     = 0;
    dZqp(1)     = 0;
    dZdn(1)     = 0;
    dZqn(1)     = 0;
    dZdz(1)     = 0;
    dZqz(1)     = 0;

end

== matlab function DQN_Lib (conflicted copy 2023-11-25 154811)/SymComp2abc_ver2/MATLAB Function ==
  data: Magp input; abc3p output; Angp input; Magn input; Angn input; Magz input; Angz input; th input; abc3n output; abc1p output; Xdp output; Xqp output; Xdn output; Xqn output; Xdz output; Xqz output
function [abc3p, abc3n ,abc1p, Xdp, Xqp, Xdn, Xqn, Xdz, Xqz] = fcn(Magp, Angp, Magn, Angn, Magz, Angz, th)

Xdp = Magp*cos(Angp);
Xqp = Magp*sin(Angp);
Xdn =-Magn*cos(Angn);
Xqn = Magn*sin(Angn);
Xdz = Magz*cos(Angz);
Xqz = Magz*sin(Angz);

Tda_p = [sin(th)            cos(th);
         sin(th-2*pi/3)     cos(th-2*pi/3);
         sin(th+2*pi/3)     cos(th+2*pi/3)];
  
Tda_n = [sin(-th)           cos(-th);
         sin(-th-2*pi/3)    cos(-th-2*pi/3);
         sin(-th+2*pi/3)    cos(-th+2*pi/3)];
  
Tda_z = [sin(th)     cos(th);
         sin(th)     cos(th);
         sin(th)     cos(th)];
     
    if(1)
        abc3p = Tda_p*[Xdp;Xqp];
        abc3n = Tda_n*[Xdn;Xqn];
        abc1p = Tda_z*[Xdz;Xqz];
    else
        Tdqn_a = [Tda_p(:,1)  Tda_n(:,1)  Tda_z(:,1)  Tda_p(:,2)  Tda_n(:,2)  Tda_z(:,2)];
        abc3p =   Tdqn_a*[Xdp;Xdn;Xdz;Xqp;Xqn;Xqz];
        abc3n = zeros(3,1);
        abc1p = zeros(3,1);
    end
end
                 
                 
% abc3n = [sin(-th)*Xdn          + cos(-th)*Xqn;
%          sin(-th-2*pi/3)*Xdn   + cos(-th-2*pi/3)*Xqn;
%          sin(-th+2*pi/3)*Xdn   + cos(-th+2*pi/3)*Xqn];
% 
% abc1p = [sin(th)*Xdz           + cos(th)*Xqz;
%          sin(th-0*2*pi/3)*Xdz  + cos(th-0*2*pi/3)*Xqz;
%          sin(th+0*2*pi/3)*Xdz  + cos(th+0*2*pi/3)*Xqz];  

% 
% abc3p = [sin(th)*Xdp           + cos(th)*Xqp;
%          sin(th-2*pi/3)*Xdp    + cos(th-2*pi/3)*Xqp;
%          sin(th+2*pi/3)*Xdp    + cos(th+2*pi/3)*Xqp];
%                  
%                  
% abc3n = [sin(-th)*Xdn          + cos(-th)*Xqn;
%          sin(-th-2*pi/3)*Xdn   + cos(-th-2*pi/3)*Xqn;
%          sin(-th+2*pi/3)*Xdn   + cos(-th+2*pi/3)*Xqn];
% 
% abc1p = [sin(th)*Xdz           + cos(th)*Xqz;
%          sin(th-0*2*pi/3)*Xdz  + cos(th-0*2*pi/3)*Xqz;
%          sin(th+0*2*pi/3)*Xdz  + cos(th+0*2*pi/3)*Xqz];

== matlab function DQN_Lib (conflicted copy 2023-11-25 154811)/abc-->DQN/MATLAB Function ==
  settings: updateMethod=DISCRETE
  data: abc input; Ydc_dqn output
function Ydc_dqn  = fcn(abc)
    
    Ydc_dqn = zeros(6,1);
    Xdc_abc = zeros(1,3);
    
    persistent min_a;     if(isempty(min_a))  min_a   = realmax; end
    persistent min_b;     if(isempty(min_b))  min_b   = realmax; end
    persistent min_c;     if(isempty(min_c))  min_c   = realmax; end
    
    persistent max_a;     if(isempty(max_a))  max_a   = realmin; end
    persistent max_b;     if(isempty(max_b))  max_b   = realmin; end
    persistent max_c;     if(isempty(max_c))  max_c   = realmin; end


    if(abc(1)<min_a) min_a=abc(1); end;
    if(abc(2)<min_b) min_b=abc(2); end;
    if(abc(3)<min_c) min_c=abc(3); end;
    
    if(abc(1)>max_a) max_a=abc(1); end
    if(abc(2)>max_b) max_b=abc(2); end
    if(abc(3)>max_c) max_c=abc(3); end
    
    Xdc_abc = [(max_a+min_a)/2, (max_b+min_b)/2, (max_c+min_c)/2];
    Xdc_abc = Xdc_abc - sum(Xdc_abc)/3;

    
    Tad_p = (2/3)*[sin(0) sin(0-2*pi/3) sin(0+2*pi/3);  
                   cos(0) cos(0-2*pi/3) cos(0+2*pi/3);];

    Tad_z = (1/3)*[0 0 0;  
                   1 1 1;];                  

    Ta_dqn = [Tad_p(1,:); Tad_p(1,:); Tad_z(1,:); Tad_p(2,:); Tad_p(2,:); Tad_z(2,:)];

    Ydc_dqn = Ta_dqn*Xdc_abc';

end

== matlab function DQN_Lib (conflicted copy 2023-11-25 154811)/DQN Mux ==
  data: u input; y output; N parameter
function y = MUX_vec(u, N)

    y = zeros((N+1)*6,1);

    for i = 1 : (N+1)*6


        if(i <= 1*(N+1)) %dp
            y(i) = u(mod(i+N,N+1)*6+1);
        elseif(i > 1*(N+1) && i <= 2*(N+1))
            y(i) = u(mod(i+N,N+1)*6+2);
        elseif(i > 2*(N+1) && i <= 3*(N+1))
            y(i) = u(mod(i+N,N+1)*6+3);
        elseif(i > 3*(N+1) && i <= 4*(N+1))
            y(i) = u(mod(i+N,N+1)*6+4);
        elseif(i > 4*(N+1) && i <= 5*(N+1))
            y(i) = u(mod(i+N,N+1)*6+5);
        elseif(i > 5*(N+1) && i <= 6*(N+1))
            y(i) = u(mod(i+N,N+1)*6+6);
        end
    end
    
end

== matlab function DQN_Lib (conflicted copy 2023-11-25 154811)/DQN Gain ==
  data: X input; Y output; Rvec parameter; H parameter
function Y  = Gain(X, Rvec, H)

    Y = zeros(6*(H+1),1);
    Y_DQN = zeros(1*H+1,6);
    X_DQN = reshape(X,H+1,6);

    persistent Rdqn;
    persistent Rdc;
    
    R = diag(Rvec);
    
    if(isempty(Rdqn))
        Tad_p = [0      -sqrt(1/3)   sqrt(1/3);
                (2/3)   -(1/3)      -(1/3);
                (1/3)    (1/3)       (1/3)];

        Tda_p = [-0           1     1;
                 -sqrt(3/4)  -0.5   1;
                  sqrt(3/4)  -0.5   1;];
        Rdq = Tad_p*R*Tda_p;
        Rdqn = [ Rdq(3,3)	-Rdq(3,2)	 Rdq(3,2)	 0          -Rdq(3,1)	 Rdq(3,1);
                -Rdq(3,2)	 Rdq(3,3)	-Rdq(3,2)	-Rdq(3,1)	 0           Rdq(3,1);
                 Rdq(3,2)	-Rdq(3,2)	 Rdq(3,3)	-Rdq(3,1)	 Rdq(3,1)	 0;
                 0          -Rdq(3,1)	-Rdq(3,1)	 Rdq(3,3)	 Rdq(3,2)	 Rdq(3,2);
                -Rdq(3,1)	 0           Rdq(3,1)	 Rdq(3,2)	 Rdq(3,3)	 Rdq(3,2);
                 Rdq(3,1)	 Rdq(3,1)	 0           Rdq(3,2)	 Rdq(3,2)	 Rdq(3,3);];
             
        Tdqn_a = [Tda_p(:,1)  Tda_p(:,1)  0*Tda_p(:,3)  Tda_p(:,2)  Tda_p(:,2)  2*Tda_p(:,3)]/2;
        Ta_dqn = [Tad_p(1,:); Tad_p(1,:); 0*Tad_p(3,:); Tad_p(2,:); Tad_p(2,:); Tad_p(3,:)];
        Rdc = (Ta_dqn*R*Tdqn_a);
    end

    Y_DQN(1,:)     = (Rdc*X_DQN(1,:)')';
    Y_DQN(2:end,:) = (Rdqn*X_DQN(2:end,:)')';    
    Y = reshape(Y_DQN,6*(H+1),1);
    
end


% function Y  = Gain(X, A, H)
% 
%     Y = zeros(3+6*H,1);
% 
%     for i = 1 : H
%         
%         Y(4 + (i-1)*6) = X(3+i+0*H);
%         Y(5 + (i-1)*6) = X(3+i+1*H);
%         Y(6 + (i-1)*6) = X(3+i+2*H);
%         Y(7 + (i-1)*6) = X(3+i+3*H);
%         Y(8 + (i-1)*6) = X(3+i+4*H);
%         Y(9 + (i-1)*6) = X(3+i+5*H);
% 
%         Y(4+6*(i-1):4+(i)*6-1) = A(4:end, 4:end)*Y(4+6*(i-1):4+(i)*6-1);
%         
%         X(3+i+0*H) = Y(4 + (i-1)*6);
%         X(3+i+1*H) = Y(5 + (i-1)*6);
%         X(3+i+2*H) = Y(6 + (i-1)*6);
%         X(3+i+3*H) = Y(7 + (i-1)*6);
%         X(3+i+4*H) = Y(8 + (i-1)*6);
%         X(3+i+5*H) = Y(9 + (i-1)*6);
%     end
%     
% 
% 
%     Y(1:3) = A(1:3,1:3) * X(1:3);
% 
%     Y(4:end) = X(4:end);
%     
% end

== matlab function DQN_Lib (conflicted copy 2023-11-25 154811)/MATLAB Function11 ==
  data: Xdc_abc input; Ydc_dqn output
function Ydc_dqn = fcn(Xdc_abc)

    Ydc_dqn = zeros(6,1);
    
    Tad_p = (2/3)*[sin(0) sin(0-2*pi/3) sin(0+2*pi/3);  
                   cos(0) cos(0-2*pi/3) cos(0+2*pi/3);];

    Tad_z = (1/3)*[0 0 0;  
                   1 1 1;];                  

    Ta_dqn = [Tad_p(1,:); Tad_p(1,:); Tad_z(1,:); Tad_p(2,:); Tad_p(2,:); Tad_z(2,:)];

    Ydc_dqn = Ta_dqn*Xdc_abc;
    
end
